simulink model "pulse_heating_v2_platform_v01"  (R2025b)
settings: Solver=VariableStepAuto  StartTime=0.0  StopTime=0.25  RelTol=1e-3
PreLoadFcn:
  | addpath('C:\Users\ADMIN\Documents\MATLAB\Examples\R2025b\simscapeelectrical\BatteryThermalManagementExample');
  | addpath('C:\Users\ADMIN\Documents\MATLAB\Examples\R2025b\mcb\SIUnitsExample');
  | addpath('C:\Users\ADMIN\Documents\MATLAB\Examples\R2025b\simscapeelectrical\PMSMDriveThermalExample');
  | load_system('PMSMDriveThermal');
  | set_param('PMSMDriveThermal','SimscapeLogType','none','SimscapeLogSimulationStatistics','off');
  | set_param('PMSMDriveThermal','Dirty','off');
InitFcn:
  | % === M4-02A: Clean parameter matching (MO theory PI) ===
  | addpath('C:\Users\ADMIN\Documents\MATLAB\Examples\R2025b\simscapeelectrical\BatteryThermalManagementExample');
  | addpath('C:\Users\ADMIN\Documents\MATLAB\Examples\R2025b\mcb\SIUnitsExample');
  | addpath('C:\Users\ADMIN\Documents\MATLAB\Examples\R2025b\simscapeelectrical\PMSMDriveThermalExample');
  | load_system('PMSMDriveThermal');
  | PMSMDriveThermalData;
  | mcb_pmsm_foc_qep_f28379d_SIUnit_data;
  | clearvars('all');
  | 
  | % --- Construct clean pmsm struct from PMSMDriveThermal ---
  | pmsm = struct();
  | pmsm.Rs = Rs; pmsm.Ld = Ld; pmsm.Lq = Lq; pmsm.p = N; pmsm.FluxPM = PM;
  | pmsm.J = J; pmsm.B = 2.6369e-6; pmsm.I_rated = Imax;
  | pmsm.Ke = PM*N; pmsm.Kt = 1.5*N*PM; pmsm.N_max = 60*fnom/N;
  | pmsm.PositionOffset = 0; pmsm.QEPSlits = 1000;
  | 
  | inverter.V_dc = 70; dataType = 'double';
  | pmsm.N_base = inverter.V_dc / (sqrt(3)*PM*N*2*pi/60);
  | pmsm.T_rated = 1.5*N*PM*Imax;
  | 
  | % --- Timing (PMSMDriveThermal semantics) ---
  | Ts = 2e-6; fsw = 2e3; fc = fsw*10; Tsc = 1/fc;
  | T_pwm = 1/fsw; PWM_frequency = fsw; Ts_simulink = Tsc;
  | Ts_motor = Tsc; Ts_speed = 10*Tsc; Ts_inverter = Tsc;
  | 
  | % --- PI gains via mcb.calcFOCGains (MO theory) ---
  | motor = pmsm; motor.Rs = pmsm.Rs + inverter.R_board;
  | PI_params = mcb.calcFOCGains(motor, Tsc, Ts_speed, SpdLPFltCoeff=0.01);
  | PI_params.delay_Currents = int32(1);
  | PI_params.delay_Position = int32(1);
  | 
  | BatteryThermalManagementInitialization;
  | ambient = 263.15; coolantTemp = 263.15;
  | cellT_ini = ambient*ones(1,Ns*Np); cellT_ini4 = ambient*ones(1,Ns4*Np4);
  | Ns_total = 3*Ns + Ns4; Np_total = Np;
  | R_pack = Ns_total * R0_mat(3,2) / Np_total;
  | I_base_A = AH * Np_total; V_pack_nom = Ns_total * 3.3;
  | 
  | % === M4-01 generalized Reference / Platform contract ===
  | % Values are traceable engineering/platform defaults, not device ratings.
  | ReferenceConfig_ID = 'M4-01-REF-PLATFORM-v02';
  | ReferenceConfig_Source = 'OFFICIAL+ENGINEERING_DEFAULT';
  | ReferenceConfig_Scope = 'generalized_system_integration';
  | HVPath_R = 0.01;
  | DCLink_C = 470e-6;
  | DCLink_V0 = 0;
  | RMS_Window_s = 20/fsw;
  | IGBT_Ron_ref = 1e-3;
  | IGBT_Vf_ref = 1.2;
  | 
  | % Encoder/reference topology provides the static mechanical boundary.
  | OpenLoop_Vabc_Scale = 1;
model workspace (MAT data in the model file):
  M401C_C_batt_J_K = 26000
  M401C_C_hv_J_K = 200
  M401C_C_inv_J_K = 3.06
  M401C_C_pmsm_rotor_J_K = 200
  M401C_C_pmsm_stator_J_K = 100
  M401C_Config_ID = 'M4-01C-REF-THERMAL-v01'
  M401C_IGBT_Eoff_ref_J = 0.01714
  M401C_IGBT_Eon_ref_J = 0.02286
  M401C_IGBT_Iref_A = 600
  M401C_IGBT_Ron_ref_Ohm = 0.001
  M401C_IGBT_Vf_ref_V = 0.8
  M401C_IGBT_Vscale_ref = 0.228137066667
  M401C_PMSM_initial_temperature_degC = -10
  M401C_PWM_fsw_Hz = 2000
  M401C_PWM_tdead_s = 1e-06
  M401C_R_batt_heat_ref_Ohm = 0.4198
  M401C_Rth_hv_K_W = 10
  M401C_Rth_inv_K_W = 0.0966666666667
  M401C_T_ambient_K = 263.15
  M401C_stall_speed_tol_rad_s = 1e-06
  control_status_v4d2_partial_duty_code = 6
  diagnostic_frequency_Hz = 50
  drive_status_v4d2_partial_current_code = 6
  kpi_status_v4d2_partial_numeric_code = 6
  kpi_value_unknown = nan
  limit_factor_unknown_code = 99
  limit_margin_unknown_value = nan
  limit_status_v4c_code = 5
  pulse_command_status_code = 6
  pulse_duty_percent = 50
  pulse_id_amplitude_A = 40
  pulse_iq_amplitude_A = 0
  pulse_mode_code = 4
  pulse_phase_delay_s = 0
undefined symbols (not defined in the file): a0, DiscIntNeverNeededParam, ECM_C1, ECM_C2, ECM_R0, ECM_R1, ECM_R2, f_eval, f_losses, Flowrate_vec, Isc_losses, losses_oc, losses_sc, N, PM, Rs
libraries: fl_lib x38, nesl_utility x35, ee_lib x12, mcbcontrolslib x5, mcbeeMathTransformLib x3, slpidlib x2, mcbhdlpositiondecoderlib x1, eePwmGeneratorTwoLevel x1
(part 5 of 5)

== matlab function pulse_heating_v2_platform_v01/System_Audit/Energy_And_Thermal_Audit/Compute_Reference_Thermal_Subledger_V4I ==
  data: t input double size=[1 1]; DeltaE_batt output double size=[1 1]; window_s input double size=[1 1]; V_batt input double size=[1 1]; I_batt input double size=[1 1]; P_hv_loss input double size=[1 1]; P_inv input double size=[1 1]; P_batt_heat input double size=[1 1]; P_cu input double size=[1 1]; P_iron input double size=[1 1]; T_pack_cells input double size=[42 1]; T_A input double size=[1 1]; T_B input double size=[1 1]; T_C input double size=[1 1]; T_R input double size=[1 1]; w_motor input double size=[1 1]; trq_motor input double size=[1 1]; P_dc_link_storage input double size=[1 1]; P_thermal_storage output double size=[1 1]; P_heat_rejection output double size=[1 1]; P_unmodeled output double size=[1 1]; thermal_contract_valid output double size=[1 1]; M401C_T_ambient_K parameter double size=[1 1]; M401C_Rth_hv_K_W parameter double size=[1 1]; M401C_Rth_inv_K_W parameter double size=[1 1]; M401C_C_hv_J_K parameter double size=[1 1]; M401C_C_inv_J_K parameter double size=[1 1]; M401C_C_batt_J_K parameter double size=[1 1]; M401C_C_pmsm_stator_J_K parameter double size=[1 1]; M401C_C_pmsm_rotor_J_K parameter double size=[1 1]
function [DeltaE_batt, P_thermal_storage, P_heat_rejection, P_unmodeled, thermal_contract_valid] = fcn(t, window_s, V_batt, I_batt, P_hv_loss, P_inv, P_batt_heat, P_cu, P_iron, T_pack_cells, T_A, T_B, T_C, T_R, w_motor, trq_motor, P_dc_link_storage, M401C_T_ambient_K, M401C_Rth_hv_K_W, M401C_Rth_inv_K_W, M401C_C_hv_J_K, M401C_C_inv_J_K, M401C_C_batt_J_K, M401C_C_pmsm_stator_J_K, M401C_C_pmsm_rotor_J_K)
% M4-01C fixed-window Reference thermal ledger. No product-level heat claim is implied.
persistent initialized active_window t_window_start t_prev P_chem_prev P_heat_prev P_mech_prev E_chem_int E_heat_int E_mech_int E_thermal_start E_thermal_prev T_pack_initial T_A_initial T_B_initial T_C_initial T_R_initial T_hv T_inv DeltaE_batt_latched P_thermal_storage_latched P_heat_rejection_latched P_mech_latched has_window
DeltaE_batt = NaN;
P_thermal_storage = NaN;
P_heat_rejection = NaN;
P_unmodeled = NaN;
thermal_contract_valid = 0;
if isempty(initialized)
    initialized = false;
    active_window = 0;
    t_window_start = 0;
    t_prev = 0;
    P_chem_prev = 0;
    P_heat_prev = 0;
    P_mech_prev = 0;
    E_chem_int = 0;
    E_heat_int = 0;
    E_mech_int = 0;
    E_thermal_start = 0;
    E_thermal_prev = 0;
    T_pack_initial = 0;
    T_A_initial = 0;
    T_B_initial = 0;
    T_C_initial = 0;
    T_R_initial = 0;
    T_hv = 0;
    T_inv = 0;
    DeltaE_batt_latched = NaN;
    P_thermal_storage_latched = NaN;
    P_heat_rejection_latched = NaN;
    P_mech_latched = NaN;
    has_window = false;
end
inputs_valid = ~(isnan(t) || isinf(t) || isnan(window_s) || isinf(window_s) || window_s <= 0);
inputs_valid = inputs_valid && ~(isnan(V_batt) || isinf(V_batt) || isnan(I_batt) || isinf(I_batt));
inputs_valid = inputs_valid && ~(isnan(P_hv_loss) || isinf(P_hv_loss) || isnan(P_inv) || isinf(P_inv));
inputs_valid = inputs_valid && ~(isnan(P_batt_heat) || isinf(P_batt_heat) || isnan(P_cu) || isinf(P_cu));
inputs_valid = inputs_valid && ~(isnan(P_iron) || isinf(P_iron) || isnan(w_motor) || isinf(w_motor));
inputs_valid = inputs_valid && ~(isnan(trq_motor) || isinf(trq_motor));
inputs_valid = inputs_valid && ~any(isnan(T_pack_cells(:))) && ~any(isinf(T_pack_cells(:)));
inputs_valid = inputs_valid && ~(isnan(T_A) || isinf(T_A) || isnan(T_B) || isinf(T_B));
inputs_valid = inputs_valid && ~(isnan(T_C) || isinf(T_C) || isnan(T_R) || isinf(T_R));
if inputs_valid
    T_pack = sum(T_pack_cells(:)) / numel(T_pack_cells);
    P_chem_now = V_batt * I_batt + P_batt_heat;
    P_heat_now = P_batt_heat + P_hv_loss + P_inv + P_cu + P_iron;
    P_mech_now = w_motor * trq_motor;
    if ~initialized || t < t_prev || window_s ~= active_window
        initialized = true;
        active_window = window_s;
        t_window_start = t;
        t_prev = t;
        P_chem_prev = P_chem_now;
        P_heat_prev = P_heat_now;
        P_mech_prev = P_mech_now;
        E_chem_int = 0;
        E_heat_int = 0;
        E_mech_int = 0;
        T_pack_initial = T_pack;
        T_A_initial = T_A;
        T_B_initial = T_B;
        T_C_initial = T_C;
        T_R_initial = T_R;
        T_hv = M401C_T_ambient_K;
        T_inv = M401C_T_ambient_K;
        E_thermal_start = 0;
        E_thermal_prev = 0;
        DeltaE_batt_latched = NaN;
        P_thermal_storage_latched = NaN;
        P_heat_rejection_latched = NaN;
        P_mech_latched = NaN;
        has_window = false;
    elseif t > t_prev
        dt = t - t_prev;
        P_hv_rejection = (T_hv - M401C_T_ambient_K) / M401C_Rth_hv_K_W;
        P_inv_rejection = (T_inv - M401C_T_ambient_K) / M401C_Rth_inv_K_W;
        T_hv = T_hv + dt * (P_hv_loss - P_hv_rejection) / M401C_C_hv_J_K;
        T_inv = T_inv + dt * (P_inv - P_inv_rejection) / M401C_C_inv_J_K;
        E_thermal_now = M401C_C_batt_J_K * (T_pack - T_pack_initial) + M401C_C_pmsm_stator_J_K * ((T_A - T_A_initial) + (T_B - T_B_initial) + (T_C - T_C_initial)) + M401C_C_pmsm_rotor_J_K * (T_R - T_R_initial) + M401C_C_hv_J_K * (T_hv - M401C_T_ambient_K) + M401C_C_inv_J_K * (T_inv - M401C_T_ambient_K);
        window_end = t_window_start + active_window;
        if t < window_end - 1e-9   % FP-safe boundary: accumulated window_end may drift ~1e-17 from DigitalClock grid
            E_chem_int = E_chem_int + 0.5 * (P_chem_prev + P_chem_now) * dt;
            E_heat_int = E_heat_int + 0.5 * (P_heat_prev + P_heat_now) * dt;
            E_mech_int = E_mech_int + 0.5 * (P_mech_prev + P_mech_now) * dt;
        else
            dt_total = t - t_prev;
            dt_head = window_end - t_prev;
            alpha = dt_head / dt_total;
            P_chem_boundary = P_chem_prev + alpha * (P_chem_now - P_chem_prev);
            P_heat_boundary = P_heat_prev + alpha * (P_heat_now - P_heat_prev);
            P_mech_boundary = P_mech_prev + alpha * (P_mech_now - P_mech_prev);
            E_thermal_boundary = E_thermal_prev + alpha * (E_thermal_now - E_thermal_prev);
            E_chem_int = E_chem_int + 0.5 * (P_chem_prev + P_chem_boundary) * dt_head;
            E_heat_int = E_heat_int + 0.5 * (P_heat_prev + P_heat_boundary) * dt_head;
            E_mech_int = E_mech_int + 0.5 * (P_mech_prev + P_mech_boundary) * dt_head;
            DeltaE_batt_latched = -E_chem_int;
            P_thermal_storage_latched = (E_thermal_boundary - E_thermal_start) / active_window;
            P_heat_rejection_latched = E_heat_int / active_window - P_thermal_storage_latched;
            P_mech_latched = E_mech_int / active_window;
            has_window = true;
            t_window_start = window_end;
            E_thermal_start = E_thermal_boundary;
            dt_tail = t - window_end;
            E_chem_int = 0.5 * (P_chem_boundary + P_chem_now) * dt_tail;
            E_heat_int = 0.5 * (P_heat_boundary + P_heat_now) * dt_tail;
            E_mech_int = 0.5 * (P_mech_boundary + P_mech_now) * dt_tail;
        end
        t_prev = t;
        P_chem_prev = P_chem_now;
        P_heat_prev = P_heat_now;
        P_mech_prev = P_mech_now;
        E_thermal_prev = E_thermal_now;
    end
else
    initialized = false;
    has_window = false;
end
if has_window
    DeltaE_batt = DeltaE_batt_latched;
    P_thermal_storage = P_thermal_storage_latched;
    P_heat_rejection = P_heat_rejection_latched;
    if ~(isnan(P_dc_link_storage) || isinf(P_dc_link_storage))
        P_unmodeled = -DeltaE_batt_latched / active_window - P_dc_link_storage - P_thermal_storage_latched - P_heat_rejection_latched - P_mech_latched;
        thermal_contract_valid = 1;
    end
end
end

== matlab function pulse_heating_v2_platform_v01/MCB_SIUnits_FOC_Controller/dSVPWM_Gate_Generator ==
  data: inputs input size=[6 1]; gates output size=[6 1]; fsw parameter; a0 parameter
function gates = fcn(inputs, fsw, a0)
%#codegen
% dSVPWM Gate Generator (M5-02)
% inputs: [Vabc(3); Vdc; bn; t] = 6x1
% gates: 6x1

gates = zeros(6, 1);
Vabc = inputs(1:3);
Vdc = inputs(4);
bn = inputs(5);
t_sim = inputs(6);
Tsw = 1.0 / fsw;

Va = Vabc(1); Vb = Vabc(2); Vc = Vabc(3);
Valpha = Va - 0.5*Vb - 0.5*Vc;
Vbeta = (sqrt(3.0)/2.0)*(Vb - Vc);

theta = atan2(Vbeta, Valpha);
if theta < 0
    theta = theta + 2.0*pi;
end
theta_deg = theta * 180.0/pi;
sector = floor(theta_deg / 60.0) + 1;
if sector > 6
    sector = 6;
end
if sector < 1
    sector = 1;
end
theta_local_deg = theta_deg - double(sector-1)*60.0;
theta_local = theta_local_deg * pi/180.0;

v1_table = [4 6 2 3 1 5];
v2_table = [6 2 3 1 5 4];
v1 = v1_table(sector);
v2 = v2_table(sector);

Vref_mag = sqrt(Valpha*Valpha + Vbeta*Vbeta);
T1 = sqrt(3.0) * Tsw * Vref_mag * sin((60.0 - theta_local_deg)*pi/180.0) / Vdc;
T2 = sqrt(3.0) * Tsw * Vref_mag * sin(theta_local) / Vdc;
T0 = Tsw - T1 - T2;

% Overmodulation: clamp T0 to 0, degenerate to standard SVPWM
if T0 < 0
    s_val = T1 + T2;
    if s_val > 0
        T1 = T1/s_val * Tsw; T2 = Tsw - T1;
    else
        T1 = 0; T2 = 0;
    end
    T0 = 0;
    bn = 0;  % disable dSVPWM in overmodulation
end

Td = a0 * T0 * bn / (1.0 + a0);
Tc = T0 * bn / (1.0 + a0);
T0p = T0 * (1.0 - bn);

gates_table = [0 1 0 1 1 0; 0 1 1 0 0 1; 0 1 1 0 1 0; 1 0 0 1 0 1; 1 0 0 1 1 0; 1 0 1 0 0 1];
v1_state = gates_table(v1, :);
v2_state = gates_table(v2, :);
comp_state = 1 - v1_state;
u0_state = [0 1 0 1 0 1];
dead_state = [0 0 0 0 0 0];

t_mod = mod(t_sim, Tsw);

t1e = T1/2.0;
t2e = t1e + T2/2.0;
t3e = t2e + T0p/2.0;
t4e = t3e + Td/2.0;
t5e = t4e + Tc;
t6e = t5e + Td/2.0;
t7e = t6e + T0p/2.0;
t8e = t7e + T2/2.0;

if t_mod < t1e
    gates(:) = v1_state(:);
elseif t_mod < t2e
    gates(:) = v2_state(:);
elseif t_mod < t3e
    gates(:) = u0_state(:);
elseif t_mod < t4e
    gates(:) = dead_state(:);
elseif t_mod < t5e
    gates(:) = comp_state(:);
elseif t_mod < t6e
    gates(:) = dead_state(:);
elseif t_mod < t7e
    gates(:) = u0_state(:);
elseif t_mod < t8e
    gates(:) = v2_state(:);
else
    gates(:) = v1_state(:);
end
end

== matlab function pulse_heating_v2_platform_v01/System_Audit/Energy_And_Thermal_Audit/Compute_Re_Z_FreqDomain ==
  data: T_pack input size=1; Re_Z_vec output size=[7 1]; SOC input size=1; Re_Z_dc output size=1; ECM_R0 parameter; ECM_R1 parameter; ECM_C1 parameter; ECM_R2 parameter; ECM_C2 parameter; f_eval parameter
function [Re_Z_vec, Re_Z_dc] = fcn(T_pack, SOC, ECM_R0, ECM_R1, ECM_C1, ECM_R2, ECM_C2, f_eval)
%#codegen
% M5-03: Compute battery Re(Z) at evaluation frequencies
% Based on NPBH 2026 Eq.5 second-order ECM
% Inputs:
%   T_pack: scalar minimum pack temperature (K) - for future T-dependence
%   SOC: scalar SOC - for future SOC-dependence
% Outputs:
%   Re_Z_vec: [7x1] Re(Z) at each f_eval frequency
%   Re_Z_dc: scalar Re(Z) at f=0 (DC, = R0+R1+R2)

% ECM parameters (ENGINEERING_DEFAULT, from base workspace)
R0 = ECM_R0;
R1 = ECM_R1;
C1 = ECM_C1;
R2 = ECM_R2;
C2 = ECM_C2;
f_eval_local = f_eval;

% Temperature and SOC dependence: currently fixed (platform assumption)
% T_pack and SOC are accepted as inputs for future extension
% but do not modify the parameters in this version.

% Compute Re(Z) at each frequency
Nf = length(f_eval_local);
Re_Z_vec = zeros(Nf, 1);
for k = 1:Nf
    w = 2.0 * pi * f_eval_local(k);
    Re_Z_vec(k) = R0 + R1/(1.0 + w^2*R1^2*C1^2) + R2/(1.0 + w^2*R2^2*C2^2);
end

% DC resistance (f=0)
Re_Z_dc = R0 + R1 + R2;

end

== matlab function pulse_heating_v2_platform_v01/System_Audit/Energy_And_Thermal_Audit/Compute_P_batt_heat_freq ==
  data: P_batt_heat_freq output size=1; I_batt_rms input size=1; Re_Z_vec input size=[7 1]
function P_batt_heat_freq = fcn(I_batt_rms, Re_Z_vec)
%#codegen
% M5-03: Frequency-domain battery heat generation estimate
% Uses window RMS current and mean Re(Z) as simple estimate
% Q = I_rms^2 * Re(Z_eff), where Re(Z_eff) = mean(Re(Z_vec))

% Inputs:
%   I_batt_rms: scalar window RMS battery current (A)
%   Re_Z_vec: [7x1] Re(Z) at f_eval frequencies (Ohm)
% Output:
%   P_batt_heat_freq: frequency-domain heat estimate (W)

if ~isempty(Re_Z_vec)
    Re_Z_eff = mean(Re_Z_vec);
else
    Re_Z_eff = 0.05;
end

P_batt_heat_freq = I_batt_rms^2 * Re_Z_eff;

end

== matlab function pulse_heating_v2_platform_v01/System_Audit/Energy_And_Thermal_Audit/Compute_P_batt_heat_harmonic ==
  data: P_batt_heat_harmonic output size=1; freq_time_residual output size=1; I_batt input size=1; Re_Z_vec input size=[7 1]; Re_Z_dc input size=1; f_eval parameter size=[1 7]
function [P_batt_heat_harmonic, freq_time_residual] = fcn(I_batt, Re_Z_vec, Re_Z_dc, f_eval)
%#codegen
% M5-03 Path A: fixed-window direct DFT of the actual battery current.
% Window: 5000 samples at Ts=2e-6 s (10 ms).
% Heat: DC component plus selected-frequency Fourier components.

persistent buffer write_idx sample_count P_latched residual_latched
Ts = 2.0e-6;
N_WINDOW = 5000;
N_FREQ = 7;

if isempty(buffer)
    buffer = zeros(N_WINDOW, 1);
    write_idx = 1;
    sample_count = 0;
    P_latched = 0.0;
    residual_latched = 0.0;
end

buffer(write_idx) = I_batt;
write_idx = write_idx + 1;
if write_idx > N_WINDOW
    write_idx = 1;
end
sample_count = sample_count + 1;

if sample_count >= N_WINDOW
    mean_i = 0.0;
    sum_i2 = 0.0;
    for n = 1:N_WINDOW
        pos = write_idx + n - 1;
        if pos > N_WINDOW
            pos = pos - N_WINDOW;
        end
        x = buffer(pos);
        mean_i = mean_i + x;
        sum_i2 = sum_i2 + x*x;
    end
    mean_i = mean_i / N_WINDOW;
    P_harm = mean_i*mean_i*Re_Z_dc;

    for k = 1:N_FREQ
        f_k = f_eval(k);
        cos_sum = 0.0;
        sin_sum = 0.0;
        for n = 1:N_WINDOW
            pos = write_idx + n - 1;
            if pos > N_WINDOW
                pos = pos - N_WINDOW;
            end
            x = buffer(pos);
            phase = 2.0*pi*f_k*(n-1)*Ts;
            cos_sum = cos_sum + x*cos(phase);
            sin_sum = sin_sum + x*sin(phase);
        end
        amplitude = (2.0/N_WINDOW)*sqrt(cos_sum*cos_sum + sin_sum*sin_sum);
        P_harm = P_harm + 0.5*amplitude*amplitude*Re_Z_vec(k);
    end

    P_latched = P_harm;
    P_td_reference = (sum_i2/N_WINDOW)*Re_Z_dc;
    residual_latched = P_harm - P_td_reference;
    sample_count = 0;
end

P_batt_heat_harmonic = P_latched;
freq_time_residual = residual_latched;
end

== matlab function pulse_heating_v2_platform_v01/System_Audit/Energy_And_Thermal_Audit/Compute_P_batt_heat_timedomain ==
  data: I_batt input size=1; P_batt_heat_td output size=1; Re_Z_dc input size=1
function P_batt_heat_td = fcn(I_batt, Re_Z_dc)
%#codegen
% M5-03 Path B: Time-domain battery heat generation
% P = I(t)^2 * Re(Z_dc), where Re(Z_dc) = R0+R1+R2
% This is the time-domain reference for cross-checking frequency-domain estimates

% Input:
%   I_batt: scalar battery current (A)
%   Re_Z_dc: scalar Re(Z) at f=0 (Ohm) = R0+R1+R2
% Output:
%   P_batt_heat_td: instantaneous time-domain heat (W)

P_batt_heat_td = I_batt^2 * Re_Z_dc;

end

== matlab function pulse_heating_v2_platform_v01/System_Audit/Energy_And_Thermal_Audit/Compute_FreqThermal_Subledger ==
  data: P_freq_out output size=1; P_harm_out output size=1; P_td_out output size=1; P_M4_out output size=1; freq_time_res output size=1; waveform_valid output size=1; P_freq input size=1; P_harm input size=1; P_td input size=1; P_M4 input size=1; t_sim input size=1; window_s input size=1
function [P_freq_out, P_harm_out, P_td_out, P_M4_out, freq_time_res, waveform_valid] = fcn(P_freq, P_harm, P_td, P_M4, t_sim, window_s)
%#codegen
% M5-03: fixed-window thermal subledger.
% Uniform samples are accumulated and averaged at each window end.

persistent sum_freq sum_harm sum_td sum_M4 sample_count next_end
persistent P_freq_latched P_harm_latched P_td_latched P_M4_latched residual_latched
TOL = 1.0e-9;

if isempty(sum_freq)
    sum_freq = 0.0;
    sum_harm = 0.0;
    sum_td = 0.0;
    sum_M4 = 0.0;
    sample_count = 0;
    next_end = window_s;
    P_freq_latched = 0.0;
    P_harm_latched = 0.0;
    P_td_latched = 0.0;
    P_M4_latched = 0.0;
    residual_latched = 0.0;
end

if window_s > 0.0 && next_end <= 0.0
    next_end = window_s;
end

sum_freq = sum_freq + P_freq;
sum_harm = sum_harm + P_harm;
sum_td = sum_td + P_td;
sum_M4 = sum_M4 + P_M4;
sample_count = sample_count + 1;
waveform_valid = false;

if window_s > 0.0 && t_sim >= (next_end - TOL)
    if sample_count > 0
        P_freq_latched = sum_freq / sample_count;
        P_harm_latched = sum_harm / sample_count;
        P_td_latched = sum_td / sample_count;
        P_M4_latched = sum_M4 / sample_count;
        residual_latched = P_harm_latched - P_td_latched;
        waveform_valid = true;
    end
    sum_freq = 0.0;
    sum_harm = 0.0;
    sum_td = 0.0;
    sum_M4 = 0.0;
    sample_count = 0;
    next_end = next_end + window_s;
end

P_freq_out = P_freq_latched;
P_harm_out = P_harm_latched;
P_td_out = P_td_latched;
P_M4_out = P_M4_latched;
freq_time_res = residual_latched;
end

== matlab function pulse_heating_v2_platform_v01/System_Audit/Energy_And_Thermal_Audit/Compute_P_cu_V4E ==
  data: Idq_debug input; P_cu output; Rs input
function P_cu = fcn(Idq_debug, Rs)
% E1: Motor copper loss P_cu = 1.5 * Rs * (Id^2 + Iq^2)
Id_fb = Idq_debug(2);
Iq_fb = Idq_debug(4);
P_cu = 1.5 * Rs * (Id_fb^2 + Iq_fb^2);
end

== matlab function pulse_heating_v2_platform_v01/PMSMDriveThermal_Inverter_And_Motor/Scopes/losses/MATLAB Function ==
  data: i_d input; trq_loss output; i_q input; w input; PM parameter; N parameter; losses_oc parameter; losses_sc parameter; f_losses parameter; Isc_losses parameter
function trq_loss = fcn(i_d,i_q,w,PM, N, losses_oc, losses_sc, f_losses, Isc_losses)

lambda = 2*pi*PM/(sqrt(2)*N);
a_h = losses_oc(1)/f_losses;
a_J = losses_oc(2)/f_losses^2;
a_ex = losses_oc(3)/f_losses^1.5;

b_h = losses_sc(1)/f_losses;
b_J = losses_sc(2)/f_losses^2;
b_ex = losses_sc(3)/f_losses^1.5;

Id = abs(i_d)/sqrt(2);
w_abs = abs(w);
if Id>0.999*Isc_losses
    ratio_Id_Isc = 0.999;
else
    ratio_Id_Isc = Id/Isc_losses;
end
Vd = lambda*w_abs*N/(2*pi)*ratio_Id_Isc; 
Iq = abs(i_q)/sqrt(2);
Vm = lambda*w_abs*N/(2*pi)*sqrt((1-ratio_Id_Isc)^2+(Iq/Isc_losses)^2);

Vm_losses = a_h/lambda*Vm+a_J/lambda^2*Vm^2+a_ex/lambda^1.5*Vm^1.5;
Vd_losses = b_h/lambda*Vd+b_J/lambda^2*Vd^2+b_ex/lambda^1.5*Vd^1.5;

trq_loss = sign(w)*(Vd_losses+Vm_losses)/(w_abs+1);

== matlab function pulse_heating_v2_platform_v01/PMSMDriveThermal_Inverter_And_Motor/Compute_Current_KPI_V4D2 ==
  data: i_abc input; i_rms output; i_peak output
function [i_rms, i_peak] = f(i_abc)
                                  i = i_abc(:);                      
                                  i_rms = sqrt(sum(i.^2)/numel(i));  
                                  i_peak = max(abs(i));              
                                  end

== matlab function pulse_heating_v2_platform_v01/MCB_SIUnits_FOC_Controller/Compute_Duty_KPI_V4D2 ==
  data: duty_abc input; mod_index output; sat_flag output
function [mod_index, sat_flag] = f(duty_abc)
                                           d = duty_abc(:);                            
                                           mod_index = max(abs(2*d - 1));              
                                           sat_flag = double(any(d <= 0 | d >= 1));    
                                           end

== matlab function pulse_heating_v2_platform_v01/System_Audit/Energy_And_Thermal_Audit/Compute_P_iron_V4E ==
  data: trq_loss input double size=[1 1]; P_iron output double size=[1 1]; w_motor input double size=[1 1]; M401C_stall_speed_tol_rad_s parameter double size=[1 1]
function P_iron = fcn(trq_loss, w_motor, M401C_stall_speed_tol_rad_s)
% M4-01C only admits the locked-rotor Reference condition.
if isnan(trq_loss) || isinf(trq_loss) || isnan(w_motor) || isinf(w_motor)
    P_iron = NaN;
elseif abs(w_motor) <= M401C_stall_speed_tol_rad_s
    P_iron = 0;
else
    P_iron = NaN;
end
end

== matlab function pulse_heating_v2_platform_v01/System_Audit/Energy_And_Thermal_Audit/Compute_P_inv_V4E ==
  data: i_abc input double size=[3 1]; P_inv output double size=[1 1]; Ron input double size=[1 1]; Vf input double size=[1 1]; M401C_IGBT_Iref_A parameter double size=[1 1]; M401C_PWM_fsw_Hz parameter double size=[1 1]; M401C_IGBT_Eon_ref_J parameter double size=[1 1]; M401C_IGBT_Eoff_ref_J parameter double size=[1 1]; M401C_IGBT_Vscale_ref parameter double size=[1 1]; M401C_PWM_tdead_s parameter double size=[1 1]
function P_inv = fcn(i_abc, Ron, Vf, M401C_IGBT_Iref_A, M401C_PWM_fsw_Hz, M401C_IGBT_Eon_ref_J, M401C_IGBT_Eoff_ref_J, M401C_IGBT_Vscale_ref, M401C_PWM_tdead_s)
% M4-01C Reference inverter loss: conduction, scaled switching, and deadtime.
i = i_abc(:);
I_rms = sqrt(sum(i.^2) / numel(i));
I_avg = sum(abs(i)) / numel(i);
P_cond = 2 * (Vf * I_avg + Ron * I_rms^2);
current_scale = min(I_rms / M401C_IGBT_Iref_A, 1);
P_switch = 6 * M401C_PWM_fsw_Hz * (M401C_IGBT_Eon_ref_J + M401C_IGBT_Eoff_ref_J) * current_scale * M401C_IGBT_Vscale_ref;
P_deadtime = 6 * M401C_PWM_fsw_Hz * M401C_PWM_tdead_s * Vf * I_avg;
P_inv = P_cond + P_switch + P_deadtime;
end
